simulink model "oloop1t"  (Simulink 2.09)
settings: Solver=ode15s  StartTime=0.0  StopTime=120  MaxStep=2  RelTol=1e-3  AbsTol=1e-3
undefined symbols (not defined in the file or in its folder): sfunyst, uaero0, uprop0
settings Model: SaveTime=off  SaveOutput=off  ConsistencyChecking=off  RTWTemplateMakefile=grt_vc.tmf

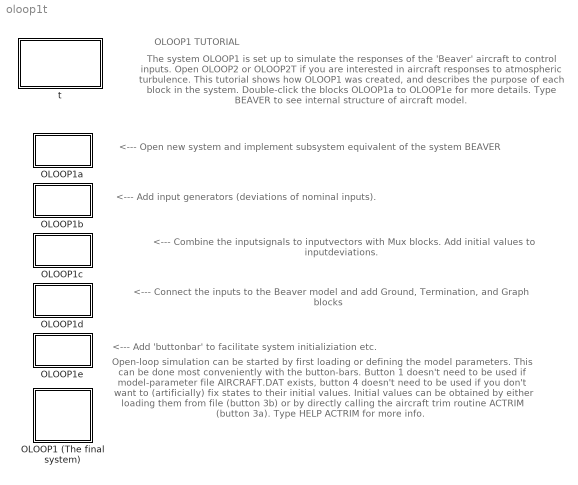
== system oloop1t ==
  note: OLOOP1 TUTORIAL
  note: <--- Connect the inputs to the Beaver model and add Ground, Termination, and Graph blocks
  note: <--- Combine the inputsignals to inputvectors with Mux blocks. Add initial values to inputdeviations.
  note: <--- Open new system and implement subsystem equivalent of the system BEAVER
  note: The system OLOOP1 is set up to simulate the responses of the 'Beaver' aircraft to control
      | inputs. Open OLOOP2 or OLOOP2T if you are interested in aircraft responses to
      | atmospheric turbulence. This tutorial shows how OLOOP1 was created, and describes
      | the purpose of each block in the system. Double-click the blocks OLOOP1a to OLOOP1e
      | for more details. Type BEAVER to see internal structure of aircraft model.
  note: <--- Add input generators (deviations of nominal inputs).
  note: Open-loop simulation can be started by first loading or defining the model parameters.
      | This can be done most conveniently with the button-bars. Button 1 doesn't need to
      | be used if model-parameter file AIRCRAFT.DAT exists, button 4 doesn't need to be
      |  used if you don't want to (artificially) fix states to their initial values. Initial values can be
      | obtained by either loading them from file (button 3b) or by directly calling the aircraft
      | trim routine ACTRIM (button 3a). Type HELP ACTRIM for more info.
  note: <--- Add 'buttonbar' to facilitate system initializiation etc.
  OLOOP1 (The final system) : Subsystem
      settings: OpenFcn=oloop1
  OLOOP1a : Subsystem
  OLOOP1b : Subsystem
  OLOOP1c : Subsystem
  OLOOP1d : Subsystem
  OLOOP1e : Subsystem
  t : Subsystem
      settings: OpenFcn=fdchelp oloop
      mask Display: disp('OLOOP1T\nMarc Rauw\nOctober 1997')

== system oloop1t/OLOOP1 (The final system) ==

== system oloop1t/OLOOP1a ==
  note: Construction of OLOOP1
  note: Step 1: open a new system
  note: Step 2: open the main FDC library FDCLIB by typing fdclib at the Matlab command-line
  note: Step 3: double-click the upper-right, light blue block (subsystem equivalents of the model BEAVER),
      | and copy the open-loop version of these subsystems to the new Simulink system
  note: Note: here a dummy version of  this
      | model has been used to reduce the
      | file-size of the tutorial
  Beaver model : Subsystem
  wires:
  Beaver model/1(V) -> ?
  Beaver model/2(alpha) -> ?
  Beaver model/3(beta) -> ?
  Beaver model/4(p) -> ?
  Beaver model/5(q) -> ?
  Beaver model/6(r) -> ?
  Beaver model/7(psi) -> ?
  Beaver model/8(theta) -> ?
  Beaver model/9(phi) -> ?
  Beaver model/10(xe) -> ?
  Beaver model/11(ye) -> ?
  Beaver model/12(H) -> ?
  Beaver model/13(H dot) -> ?
  Beaver model/14(pb/2V) -> ?
  Beaver model/15(qc/V) -> ?
  Beaver model/16(rb/2V) -> ?
  ? -> Beaver model/1(uaero)
  ? -> Beaver model/2(uprop)
  ? -> Beaver model/3(uwind)

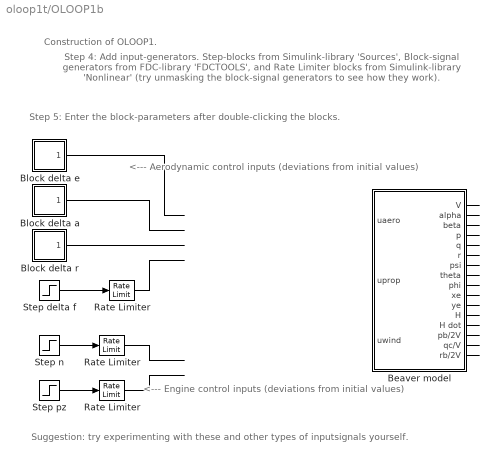
== system oloop1t/OLOOP1b ==
  note: Construction of OLOOP1.
  note: Step 5: Enter the block-parameters after double-clicking the blocks.
  note: Step 4: Add input-generators. Step-blocks from Simulink-library 'Sources', Block-signal generators
      | from FDC-library 'FDCTOOLS', and Rate Limiter blocks from Simulink-library 'Nonlinear'
      | (try unmasking the block-signal generators to see how they work).
  note: Suggestion: try experimenting with these and other types of inputsignals yourself.
  note: <--- Engine control inputs
      | (deviations from initial values)
  note: <--- Aerodynamic control inputs
      | (deviations from initial values)
  " Rate Limiter" : RateLimiter  RisingSlewLimit=1.0  FallingSlewLimit=-1.0
  Beaver model : Subsystem
  Block delta a : Subsystem  mask(Block Fcn){@1=0, @2=3*pi/180, @3=0, @4=2}
      mask prompts: @1 "Initial value (=final value):"; @2 "Amplitude of block (+ = step up, - = step down):"; @3 "Start time of block:"; @4 "Stop time of block:"
      mask help: Block Function
      mask init:
      | yinit=@1; yblock=@2; tstart=@3; tstop=@4;
      mask Help: This block implements a block signal.\nDefine the initial (=final) value, the\namplitude of the block (positive\n= upwards, negative=downwards),\nthe start time, and the stop time (must\nbe smaller than the start time).
      mask Display: plot(0,0,100,100,[100,60,60,20,20,0],[50,50,89,89,50,50])
  Block delta e : Subsystem  mask(Block Fcn){@1=0, @2=3*pi/180, @3=0, @4=2}
      mask prompts: @1 "Initial value (=final value):"; @2 "Amplitude of block (+ = step up, - = step down):"; @3 "Start time of block:"; @4 "Stop time of block:"
      mask help: Block Function
      mask init:
      | yinit=@1; yblock=@2; tstart=@3; tstop=@4;
      mask Help: This block implements a block signal.\nDefine the initial (=final) value, the\namplitude of the block (positive\n= upwards, negative=downwards),\nthe start time, and the stop time (must\nbe smaller than the start time).
      mask Display: plot(0,0,100,100,[100,60,60,20,20,0],[50,50,89,89,50,50])
  Block delta r : Subsystem  mask(Block Fcn){@1=0, @2=3*pi/180, @3=0, @4=2}
      mask prompts: @1 "Initial value (=final value):"; @2 "Amplitude of block (+ = step up, - = step down):"; @3 "Start time of block:"; @4 "Stop time of block:"
      mask help: Block Function
      mask init:
      | yinit=@1; yblock=@2; tstart=@3; tstop=@4;
      mask Help: This block implements a block signal.\nDefine the initial (=final) value, the\namplitude of the block (positive\n= upwards, negative=downwards),\nthe start time, and the stop time (must\nbe smaller than the start time).
      mask Display: plot(0,0,100,100,[100,60,60,20,20,0],[50,50,89,89,50,50])
  Rate Limiter : RateLimiter  RisingSlewLimit=3*pi/180  FallingSlewLimit=-3*pi/180
  "Rate Limiter " : RateLimiter  RisingSlewLimit=50  FallingSlewLimit=-50
  Step delta f : Step  Time=0.001  Before=0  After=3*pi/180
  Step n : Step  Time=1  Before=0  After=200
  Step pz : Step  Time=0.001  Before=0  After=2
  wires:
  Block delta a/1(block) -> ?
  Block delta r/1(block) -> ?
  Step delta f/1 -> Rate Limiter/1
  Step n/1 -> "Rate Limiter "/1
  Step pz/1 -> " Rate Limiter"/1
  Block delta e/1(block) -> ?
  Rate Limiter/1 -> ?
  "Rate Limiter "/1 -> ?
  " Rate Limiter"/1 -> ?
  Beaver model/1(V) -> ?
  Beaver model/2(alpha) -> ?
  Beaver model/3(beta) -> ?
  Beaver model/4(p) -> ?
  Beaver model/5(q) -> ?
  Beaver model/6(r) -> ?
  Beaver model/7(psi) -> ?
  Beaver model/8(theta) -> ?
  Beaver model/9(phi) -> ?
  Beaver model/10(xe) -> ?
  Beaver model/11(ye) -> ?
  Beaver model/12(H) -> ?
  Beaver model/13(H dot) -> ?
  Beaver model/14(pb/2V) -> ?
  Beaver model/15(qc/V) -> ?
  Beaver model/16(rb/2V) -> ?
  ? -> Beaver model/1(uaero)
  ? -> Beaver model/2(uprop)
  ? -> Beaver model/3(uwind)

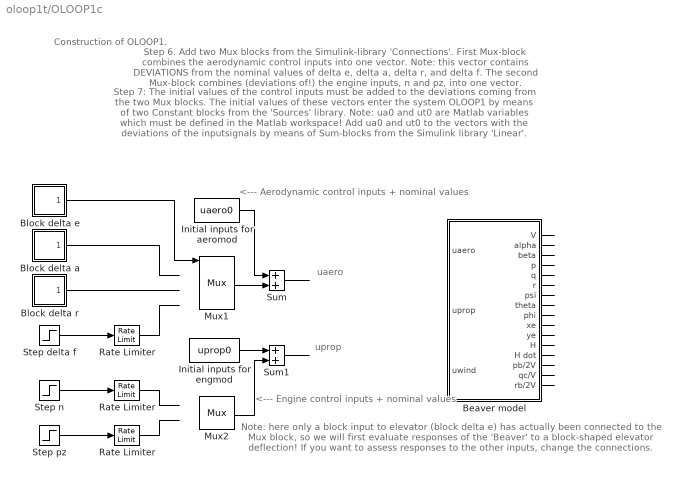
== system oloop1t/OLOOP1c ==
  note: uprop
  note: uaero
  note: Construction of OLOOP1.
  note: Note: here only a block input to elevator (block delta e) has actually
      | been connected to the Mux block, so we will first evaluate responses
      | of the 'Beaver' to a block-shaped elevator deflection! If you want to assess
      | responses to the other inputs, change the connections.
  note: <--- Aerodynamic control
      | inputs + nominal values
  note: <--- Engine control inputs +
      | nominal values
  note: Step 7: The initial values of the control inputs must be added to the deviations coming from the two Mux blocks. The initial
      | values of these vectors enter the system OLOOP1 by means of two Constant blocks from the 'Sources' library.
      | Note: ua0 and ut0 are Matlab variables which must be defined in the Matlab workspace! Add ua0 and ut0 to the
      | vectors with the deviations of the inputsignals by means of Sum-blocks from the Simulink library 'Linear'.
  note: Step 6. Add two Mux blocks from the Simulink-library 'Connections'. First Mux-block combines the aerodynamic control inputs
      | into one vector. Note: this vector contains DEVIATIONS from the nominal values of delta e, delta a, delta r, and delta f.
      | The second Mux-block combines (deviations of!) the engine inputs, n and pz, into one vector.
  " Rate Limiter" : RateLimiter  RisingSlewLimit=1.0  FallingSlewLimit=-1.0
  Beaver model : Subsystem
  Block delta a : Subsystem  mask(Block Fcn){@1=0, @2=3*pi/180, @3=0, @4=2}
      mask prompts: @1 "Initial value (=final value):"; @2 "Amplitude of block (+ = step up, - = step down):"; @3 "Start time of block:"; @4 "Stop time of block:"
      mask help: Block Function
      mask init:
      | yinit=@1; yblock=@2; tstart=@3; tstop=@4;
      mask Help: This block implements a block signal.\nDefine the initial (=final) value, the\namplitude of the block (positive\n= upwards, negative=downwards),\nthe start time, and the stop time (must\nbe smaller than the start time).
      mask Display: plot(0,0,100,100,[100,60,60,20,20,0],[50,50,89,89,50,50])
  Block delta e : Subsystem  mask(Block Fcn){@1=0, @2=3*pi/180, @3=0, @4=2}
      mask prompts: @1 "Initial value (=final value):"; @2 "Amplitude of block (+ = step up, - = step down):"; @3 "Start time of block:"; @4 "Stop time of block:"
      mask help: Block Function
      mask init:
      | yinit=@1; yblock=@2; tstart=@3; tstop=@4;
      mask Help: This block implements a block signal.\nDefine the initial (=final) value, the\namplitude of the block (positive\n= upwards, negative=downwards),\nthe start time, and the stop time (must\nbe smaller than the start time).
      mask Display: plot(0,0,100,100,[100,60,60,20,20,0],[50,50,89,89,50,50])
  Block delta r : Subsystem  mask(Block Fcn){@1=0, @2=3*pi/180, @3=0, @4=2}
      mask prompts: @1 "Initial value (=final value):"; @2 "Amplitude of block (+ = step up, - = step down):"; @3 "Start time of block:"; @4 "Stop time of block:"
      mask help: Block Function
      mask init:
      | yinit=@1; yblock=@2; tstart=@3; tstop=@4;
      mask Help: This block implements a block signal.\nDefine the initial (=final) value, the\namplitude of the block (positive\n= upwards, negative=downwards),\nthe start time, and the stop time (must\nbe smaller than the start time).
      mask Display: plot(0,0,100,100,[100,60,60,20,20,0],[50,50,89,89,50,50])
  Initial inputs for aeromod : Constant  Value=uaero0
  Initial inputs for engmod : Constant  Value=uprop0
  Mux1 : Mux  Inputs=4
  Mux2 : Mux  Inputs=2
  Rate Limiter : RateLimiter  RisingSlewLimit=3*pi/180  FallingSlewLimit=-3*pi/180
  "Rate Limiter " : RateLimiter  RisingSlewLimit=50  FallingSlewLimit=-50
  Step delta f : Step  Time=0.001  Before=0  After=3*pi/180
  Step n : Step  Time=1  Before=0  After=200
  Step pz : Step  Time=0.001  Before=0  After=2
  Sum : Sum  Inputs=++
  Sum1 : Sum  Inputs=++
  wires:
  Sum1/1 -> ?
  Sum/1 -> ?
  " Rate Limiter"/1 -> ?
  "Rate Limiter "/1 -> ?
  Rate Limiter/1 -> ?
  Block delta e/1(block) -> Mux1/1
  Step pz/1 -> " Rate Limiter"/1
  Step n/1 -> "Rate Limiter "/1
  Mux2/1 -> Sum1/2
  Mux1/1 -> Sum/2
  Initial inputs for aeromod/1 -> Sum/1
  Step delta f/1 -> Rate Limiter/1
  Initial inputs for engmod/1 -> Sum1/1
  Block delta r/1(block) -> ?
  Block delta a/1(block) -> ?
  Beaver model/2(alpha) -> ?
  Beaver model/3(beta) -> ?
  Beaver model/4(p) -> ?
  Beaver model/5(q) -> ?
  Beaver model/6(r) -> ?
  Beaver model/7(psi) -> ?
  Beaver model/8(theta) -> ?
  Beaver model/9(phi) -> ?
  Beaver model/10(xe) -> ?
  Beaver model/11(ye) -> ?
  Beaver model/12(H) -> ?
  Beaver model/13(H dot) -> ?
  Beaver model/14(pb/2V) -> ?
  Beaver model/15(qc/V) -> ?
  Beaver model/16(rb/2V) -> ?
  ? -> Beaver model/1(uaero)
  ? -> Beaver model/2(uprop)
  ? -> Beaver model/3(uwind)
  Beaver model/1(V) -> ?

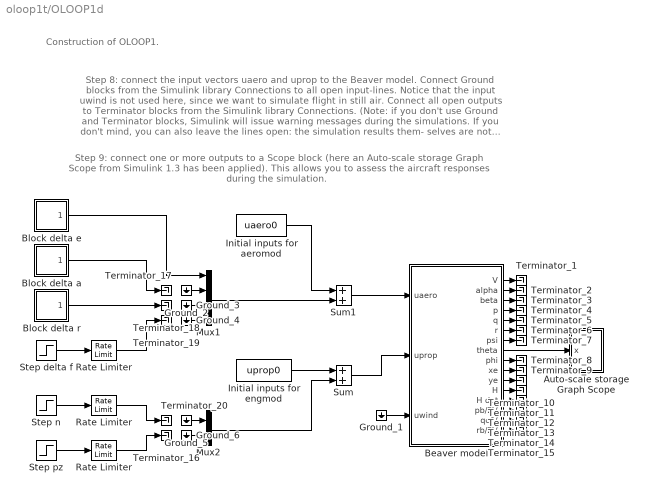
== system oloop1t/OLOOP1d ==
  note: Construction of OLOOP1.
  note: Step 9: connect one or more outputs to a Scope block (here an Auto-scale storage Graph Scope from
      | Simulink 1.3 has been applied). This allows you to assess the aircraft responses during the simulation.
  note: Step 8: connect the input vectors uaero and uprop to the Beaver model. Connect Ground blocks from the
      | Simulink library Connections to all open input-lines. Notice that the input uwind is not used here, since we
      | want to simulate flight in still air. Connect all open outputs to Terminator blocks from the Simulink library
      | Connections. (Note: if you don't use Ground and Terminator blocks, Simulink will issue warning messages
      | during the simulations. If you don't mind, you can also leave the lines open: the simulation results them-
      | selves are not affected by these warning messages).
  " Rate Limiter" : RateLimiter  RisingSlewLimit=1.0  FallingSlewLimit=-1.0
  Auto-scale storage Graph Scope : Subsystem  mask(Storage scope.){@1=5, @2=-0.02, @3=0.02, @4=200, @5='r-'}
      mask prompts: @1 "Initial Time Range:"; @2 "Initial y-min:"; @3 "Initial y-max:"; @4 "Storage pts.:"; @5 "Line type (rgbw-.:xo):"
      mask help:
      | Storage scope using MATLAB graph window.
      | Enter plotting ranges and line type.
      mask init:
      | npts = @4; color = @5; ax = [0, @1, @2, @3];
      mask Help: Uses MATLAB's graph window.\nUse only one block per system.\nLine type must be in quotes.\nSee the M-file sfunyst.m.
      mask Display: plot(0,0,100,100,[83,76,63,52,42,38,28,16,11,84,11,11,11,90,90,11],[75,58,47,54,72,80,84,74,65,65,65,90,40,40,90,90])
  Beaver model : Subsystem
  Block delta a : Subsystem  mask(Block Fcn){@1=0, @2=3*pi/180, @3=0, @4=2}
      mask prompts: @1 "Initial value (=final value):"; @2 "Amplitude of block (+ = step up, - = step down):"; @3 "Start time of block:"; @4 "Stop time of block:"
      mask help: Block Function
      mask init:
      | yinit=@1; yblock=@2; tstart=@3; tstop=@4;
      mask Help: This block implements a block signal.\nDefine the initial (=final) value, the\namplitude of the block (positive\n= upwards, negative=downwards),\nthe start time, and the stop time (must\nbe smaller than the start time).
      mask Display: plot(0,0,100,100,[100,60,60,20,20,0],[50,50,89,89,50,50])
  Block delta e : Subsystem  mask(Block Fcn){@1=0, @2=3*pi/180, @3=0, @4=2}
      mask prompts: @1 "Initial value (=final value):"; @2 "Amplitude of block (+ = step up, - = step down):"; @3 "Start time of block:"; @4 "Stop time of block:"
      mask help: Block Function
      mask init:
      | yinit=@1; yblock=@2; tstart=@3; tstop=@4;
      mask Help: This block implements a block signal.\nDefine the initial (=final) value, the\namplitude of the block (positive\n= upwards, negative=downwards),\nthe start time, and the stop time (must\nbe smaller than the start time).
      mask Display: plot(0,0,100,100,[100,60,60,20,20,0],[50,50,89,89,50,50])
  Block delta r : Subsystem  mask(Block Fcn){@1=0, @2=3*pi/180, @3=0, @4=2}
      mask prompts: @1 "Initial value (=final value):"; @2 "Amplitude of block (+ = step up, - = step down):"; @3 "Start time of block:"; @4 "Stop time of block:"
      mask help: Block Function
      mask init:
      | yinit=@1; yblock=@2; tstart=@3; tstop=@4;
      mask Help: This block implements a block signal.\nDefine the initial (=final) value, the\namplitude of the block (positive\n= upwards, negative=downwards),\nthe start time, and the stop time (must\nbe smaller than the start time).
      mask Display: plot(0,0,100,100,[100,60,60,20,20,0],[50,50,89,89,50,50])
  Ground_{1..6} (6 alike) : Ground
  Initial inputs for aeromod : Constant  Value=uaero0
  Initial inputs for engmod : Constant  Value=uprop0
  Mux1 : Mux  Inputs=4
  Mux2 : Mux  Inputs=2
  Rate Limiter : RateLimiter  RisingSlewLimit=3*pi/180  FallingSlewLimit=-3*pi/180
  "Rate Limiter " : RateLimiter  RisingSlewLimit=50  FallingSlewLimit=-50
  Step delta f : Step  Time=0.001  Before=0  After=3*pi/180
  Step n : Step  Time=1  Before=0  After=200
  Step pz : Step  Time=0.001  Before=0  After=2
  Sum : Sum  Inputs=++
  Sum1 : Sum  Inputs=++
  Terminator_{1..20} (20 alike) : Terminator
  wires:
  Beaver model/16(rb/2V) -> Terminator_15/1
  Beaver model/15(qc/V) -> Terminator_14/1
  Beaver model/14(pb/2V) -> Terminator_13/1
  Beaver model/13(H dot) -> Terminator_12/1
  Beaver model/12(H) -> Terminator_11/1
  Beaver model/11(ye) -> Terminator_10/1
  Beaver model/10(xe) -> Terminator_9/1
  Beaver model/9(phi) -> Terminator_8/1
  Beaver model/7(psi) -> Terminator_7/1
  Beaver model/6(r) -> Terminator_6/1
  Beaver model/5(q) -> Terminator_5/1
  Beaver model/4(p) -> Terminator_4/1
  Beaver model/3(beta) -> Terminator_3/1
  Beaver model/2(alpha) -> Terminator_2/1
  Beaver model/1(V) -> Terminator_1/1
  Mux2/1 -> Sum/2
  Initial inputs for aeromod/1 -> Sum1/1
  Sum/1 -> Beaver model/2(uprop)
  Initial inputs for engmod/1 -> Sum/1
  Sum1/1 -> Beaver model/1(uaero)
  Mux1/1 -> Sum1/2
  Ground_1/1 -> Beaver model/3(uwind)
  Block delta e/1(block) -> Mux1/1
  Step pz/1 -> " Rate Limiter"/1
  Step n/1 -> "Rate Limiter "/1
  Step delta f/1 -> Rate Limiter/1
  Ground_2/1 -> Mux1/2
  Ground_3/1 -> Mux1/3
  Ground_4/1 -> Mux1/4
  Ground_5/1 -> Mux2/1
  Ground_6/1 -> Mux2/2
  " Rate Limiter"/1 -> Terminator_16/1
  Block delta a/1(block) -> Terminator_17/1
  Block delta r/1(block) -> Terminator_18/1
  Rate Limiter/1 -> Terminator_19/1
  "Rate Limiter "/1 -> Terminator_20/1
  Beaver model/8(theta) -> Auto-scale storage Graph Scope/1(x)

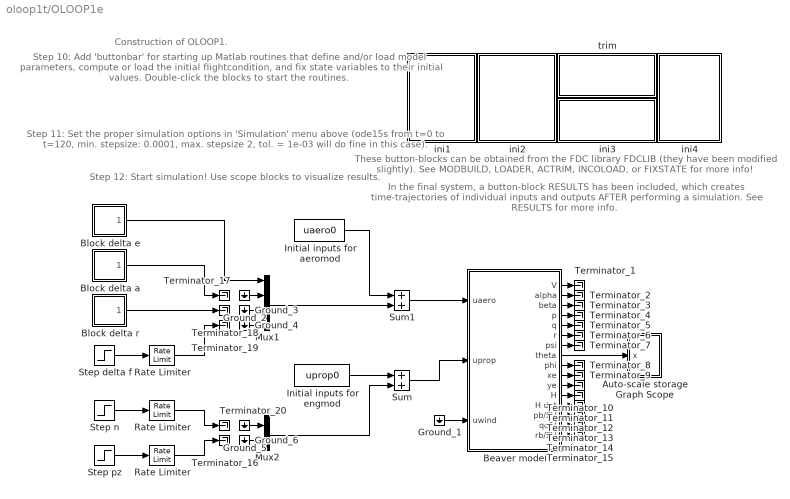
== system oloop1t/OLOOP1e ==
  note: Construction of OLOOP1.
  note: In the final system, a button-block RESULTS has been included,
      | which creates time-trajectories of individual inputs and outputs
      | AFTER performing a simulation. See RESULTS for more info.
  note: Step 11: Set the proper simulation options in 'Simulation' menu
      | above (ode15s from t=0 to t=120, min. stepsize: 0.0001,
      | max. stepsize 2, tol. = 1e-03 will do fine in this case).
  note: Step 12: Start simulation! Use scope blocks to visualize results.
  note: Step 10: Add 'buttonbar' for starting up Matlab routines that
      | define and/or load model parameters, compute or load the
      | initial flightcondition, and fix state variables to their initial
      | values. Double-click the blocks to start the routines.
  note: These button-blocks can be obtained from the FDC library
      | FDCLIB (they have been modified slightly). See MODBUILD,
      | LOADER, ACTRIM, INCOLOAD, or FIXSTATE for more info!
  " Rate Limiter" : RateLimiter  RisingSlewLimit=1.0  FallingSlewLimit=-1.0
  Auto-scale storage Graph Scope : Subsystem  mask(Storage scope.){@1=5, @2=-0.02, @3=0.02, @4=200, @5='r-'}
      mask prompts: @1 "Initial Time Range:"; @2 "Initial y-min:"; @3 "Initial y-max:"; @4 "Storage pts.:"; @5 "Line type (rgbw-.:xo):"
      mask help:
      | Storage scope using MATLAB graph window.
      | Enter plotting ranges and line type.
      mask init:
      | npts = @4; color = @5; ax = [0, @1, @2, @3];
      mask Help: Uses MATLAB's graph window.\nUse only one block per system.\nLine type must be in quotes.\nSee the M-file sfunyst.m.
      mask Display: plot(0,0,100,100,[83,76,63,52,42,38,28,16,11,84,11,11,11,90,90,11],[75,58,47,54,72,80,84,74,65,65,65,90,40,40,90,90])
  Beaver model : Subsystem
  Block delta a : Subsystem  mask(Block Fcn){@1=0, @2=3*pi/180, @3=0, @4=2}
      mask prompts: @1 "Initial value (=final value):"; @2 "Amplitude of block (+ = step up, - = step down):"; @3 "Start time of block:"; @4 "Stop time of block:"
      mask help: Block Function
      mask init:
      | yinit=@1; yblock=@2; tstart=@3; tstop=@4;
      mask Help: This block implements a block signal.\nDefine the initial (=final) value, the\namplitude of the block (positive\n= upwards, negative=downwards),\nthe start time, and the stop time (must\nbe smaller than the start time).
      mask Display: plot(0,0,100,100,[100,60,60,20,20,0],[50,50,89,89,50,50])
  Block delta e : Subsystem  mask(Block Fcn){@1=0, @2=3*pi/180, @3=0, @4=2}
      mask prompts: @1 "Initial value (=final value):"; @2 "Amplitude of block (+ = step up, - = step down):"; @3 "Start time of block:"; @4 "Stop time of block:"
      mask help: Block Function
      mask init:
      | yinit=@1; yblock=@2; tstart=@3; tstop=@4;
      mask Help: This block implements a block signal.\nDefine the initial (=final) value, the\namplitude of the block (positive\n= upwards, negative=downwards),\nthe start time, and the stop time (must\nbe smaller than the start time).
      mask Display: plot(0,0,100,100,[100,60,60,20,20,0],[50,50,89,89,50,50])
  Block delta r : Subsystem  mask(Block Fcn){@1=0, @2=3*pi/180, @3=0, @4=2}
      mask prompts: @1 "Initial value (=final value):"; @2 "Amplitude of block (+ = step up, - = step down):"; @3 "Start time of block:"; @4 "Stop time of block:"
      mask help: Block Function
      mask init:
      | yinit=@1; yblock=@2; tstart=@3; tstop=@4;
      mask Help: This block implements a block signal.\nDefine the initial (=final) value, the\namplitude of the block (positive\n= upwards, negative=downwards),\nthe start time, and the stop time (must\nbe smaller than the start time).
      mask Display: plot(0,0,100,100,[100,60,60,20,20,0],[50,50,89,89,50,50])
  Ground_{1..6} (6 alike) : Ground
  Initial inputs for aeromod : Constant  Value=uaero0
  Initial inputs for engmod : Constant  Value=uprop0
  Mux1 : Mux  Inputs=4
  Mux2 : Mux  Inputs=2
  Rate Limiter : RateLimiter  RisingSlewLimit=3*pi/180  FallingSlewLimit=-3*pi/180
  "Rate Limiter " : RateLimiter  RisingSlewLimit=50  FallingSlewLimit=-50
  Step delta f : Step  Time=0.001  Before=0  After=3*pi/180
  Step n : Step  Time=1  Before=0  After=200
  Step pz : Step  Time=0.001  Before=0  After=2
  Sum : Sum  Inputs=++
  Sum1 : Sum  Inputs=++
  Terminator_{1..20} (20 alike) : Terminator
  ini1 : Subsystem
      settings: OpenFcn=modbuild
      mask Type: modbuild
      mask Display: disp('(1). Create\ndatafiles\n\n\nMODBUILD')
  ini2 : Subsystem
      settings: OpenFcn=loader
      mask Type: loader
      mask Display: disp('2. Load model\nparameters\nfrom file\n\nLOADER')
  ini3 : Subsystem
      settings: OpenFcn=incoload
      mask Type: incoload
      mask Display: disp('3b. Load initial\ncondition from file\nINCOLOAD')
  ini4 : Subsystem
      settings: OpenFcn=fixstate
      mask Type: fixstate
      mask Display: disp('(4). Fix\nindividual\nstates\n\nFIXSTATE')
  trim : Subsystem
      settings: OpenFcn=actrim
      mask Type: aircraft trim
      mask Display: disp('3a. Call aircraft\ntrim routine\nACTRIM')
  wires:
  Beaver model/16(rb/2V) -> Terminator_15/1
  Beaver model/15(qc/V) -> Terminator_14/1
  Beaver model/14(pb/2V) -> Terminator_13/1
  Beaver model/13(H dot) -> Terminator_12/1
  Beaver model/12(H) -> Terminator_11/1
  Beaver model/11(ye) -> Terminator_10/1
  Beaver model/10(xe) -> Terminator_9/1
  Beaver model/9(phi) -> Terminator_8/1
  Beaver model/7(psi) -> Terminator_7/1
  Beaver model/6(r) -> Terminator_6/1
  Beaver model/5(q) -> Terminator_5/1
  Beaver model/4(p) -> Terminator_4/1
  Beaver model/3(beta) -> Terminator_3/1
  Beaver model/2(alpha) -> Terminator_2/1
  Beaver model/1(V) -> Terminator_1/1
  Mux2/1 -> Sum/2
  Initial inputs for aeromod/1 -> Sum1/1
  Sum/1 -> Beaver model/2(uprop)
  Initial inputs for engmod/1 -> Sum/1
  Sum1/1 -> Beaver model/1(uaero)
  Mux1/1 -> Sum1/2
  Ground_1/1 -> Beaver model/3(uwind)
  Block delta e/1(block) -> Mux1/1
  Step pz/1 -> " Rate Limiter"/1
  Step n/1 -> "Rate Limiter "/1
  Step delta f/1 -> Rate Limiter/1
  Ground_2/1 -> Mux1/2
  Ground_3/1 -> Mux1/3
  Ground_4/1 -> Mux1/4
  Ground_5/1 -> Mux2/1
  Ground_6/1 -> Mux2/2
  " Rate Limiter"/1 -> Terminator_16/1
  Block delta a/1(block) -> Terminator_17/1
  Block delta r/1(block) -> Terminator_18/1
  Rate Limiter/1 -> Terminator_19/1
  "Rate Limiter "/1 -> Terminator_20/1
  Beaver model/8(theta) -> Auto-scale storage Graph Scope/1(x)

== system oloop1t/t ==

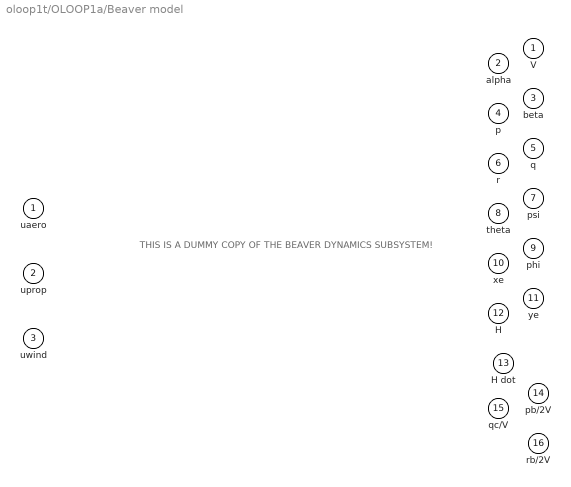
== system oloop1t/OLOOP1a/Beaver model ==
  note: THIS IS A DUMMY COPY
      | OF THE BEAVER
      | DYNAMICS SUBSYSTEM!
  uaero : Inport  Port=1  PortWidth=4  SampleTime=-1
  uprop : Inport  Port=2  PortWidth=2  SampleTime=-1
  uwind : Inport  Port=3  PortWidth=6  SampleTime=-1
  V : Outport  Port=1  InitialOutput=0
  alpha : Outport  Port=2  InitialOutput=0
  beta : Outport  Port=3  InitialOutput=0
  p : Outport  Port=4  InitialOutput=0
  q : Outport  Port=5  InitialOutput=0
  r : Outport  Port=6  InitialOutput=0
  psi : Outport  Port=7  InitialOutput=0
  theta : Outport  Port=8  InitialOutput=0
  phi : Outport  Port=9  InitialOutput=0
  xe : Outport  Port=10  InitialOutput=0
  ye : Outport  Port=11  InitialOutput=0
  H : Outport  Port=12  InitialOutput=0
  H dot : Outport  Port=13  InitialOutput=0
  pb/2V : Outport  Port=14  InitialOutput=0
  qc/V : Outport  Port=15  InitialOutput=0
  rb/2V : Outport  Port=16  InitialOutput=0

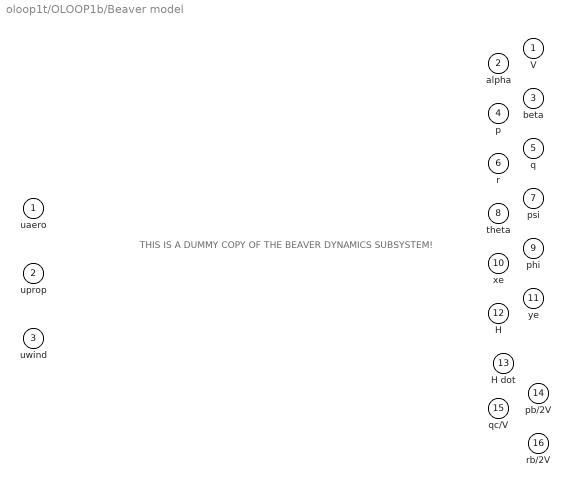
== system oloop1t/OLOOP1b/Beaver model ==
  note: THIS IS A DUMMY COPY
      | OF THE BEAVER
      | DYNAMICS SUBSYSTEM!
  uaero : Inport  Port=1  PortWidth=4  SampleTime=-1
  uprop : Inport  Port=2  PortWidth=2  SampleTime=-1
  uwind : Inport  Port=3  PortWidth=6  SampleTime=-1
  V : Outport  Port=1  InitialOutput=0
  alpha : Outport  Port=2  InitialOutput=0
  beta : Outport  Port=3  InitialOutput=0
  p : Outport  Port=4  InitialOutput=0
  q : Outport  Port=5  InitialOutput=0
  r : Outport  Port=6  InitialOutput=0
  psi : Outport  Port=7  InitialOutput=0
  theta : Outport  Port=8  InitialOutput=0
  phi : Outport  Port=9  InitialOutput=0
  xe : Outport  Port=10  InitialOutput=0
  ye : Outport  Port=11  InitialOutput=0
  H : Outport  Port=12  InitialOutput=0
  H dot : Outport  Port=13  InitialOutput=0
  pb/2V : Outport  Port=14  InitialOutput=0
  qc/V : Outport  Port=15  InitialOutput=0
  rb/2V : Outport  Port=16  InitialOutput=0

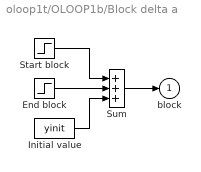
== system oloop1t/OLOOP1b/Block delta a ==
  End block : Step  Time=tstop  Before=0  After=-yblock
  Initial value : Constant  Value=yinit
  Start block : Step  Time=tstart  Before=0  After=yblock
  Sum : Sum  Inputs=+++
  block : Outport  Port=1  InitialOutput=0
  wires:
  Sum/1 -> block/1
  Initial value/1 -> Sum/3
  Start block/1 -> Sum/1
  End block/1 -> Sum/2

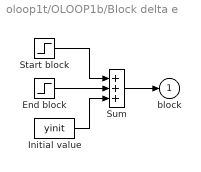
== system oloop1t/OLOOP1b/Block delta e ==
  End block : Step  Time=tstop  Before=0  After=-yblock
  Initial value : Constant  Value=yinit
  Start block : Step  Time=tstart  Before=0  After=yblock
  Sum : Sum  Inputs=+++
  block : Outport  Port=1  InitialOutput=0
  wires:
  End block/1 -> Sum/2
  Start block/1 -> Sum/1
  Initial value/1 -> Sum/3
  Sum/1 -> block/1

== system oloop1t/OLOOP1b/Block delta r ==
  End block : Step  Time=tstop  Before=0  After=-yblock
  Initial value : Constant  Value=yinit
  Start block : Step  Time=tstart  Before=0  After=yblock
  Sum : Sum  Inputs=+++
  block : Outport  Port=1  InitialOutput=0
  wires:
  End block/1 -> Sum/2
  Start block/1 -> Sum/1
  Initial value/1 -> Sum/3
  Sum/1 -> block/1

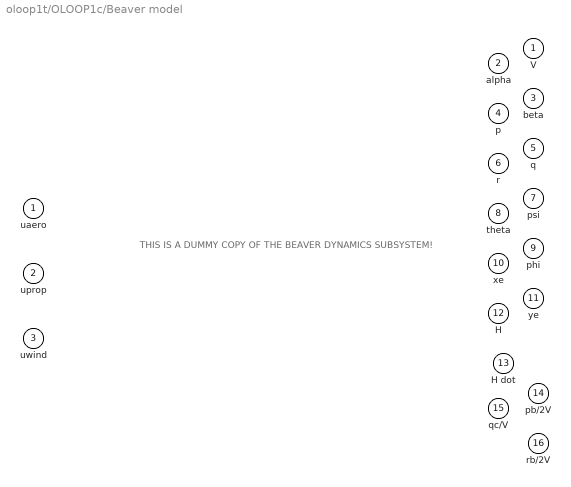
== system oloop1t/OLOOP1c/Beaver model ==
  note: THIS IS A DUMMY COPY
      | OF THE BEAVER
      | DYNAMICS SUBSYSTEM!
  uaero : Inport  Port=1  PortWidth=4  SampleTime=-1
  uprop : Inport  Port=2  PortWidth=2  SampleTime=-1
  uwind : Inport  Port=3  PortWidth=6  SampleTime=-1
  V : Outport  Port=1  InitialOutput=0
  alpha : Outport  Port=2  InitialOutput=0
  beta : Outport  Port=3  InitialOutput=0
  p : Outport  Port=4  InitialOutput=0
  q : Outport  Port=5  InitialOutput=0
  r : Outport  Port=6  InitialOutput=0
  psi : Outport  Port=7  InitialOutput=0
  theta : Outport  Port=8  InitialOutput=0
  phi : Outport  Port=9  InitialOutput=0
  xe : Outport  Port=10  InitialOutput=0
  ye : Outport  Port=11  InitialOutput=0
  H : Outport  Port=12  InitialOutput=0
  H dot : Outport  Port=13  InitialOutput=0
  pb/2V : Outport  Port=14  InitialOutput=0
  qc/V : Outport  Port=15  InitialOutput=0
  rb/2V : Outport  Port=16  InitialOutput=0

== system oloop1t/OLOOP1c/Block delta a ==
  End block : Step  Time=tstop  Before=0  After=-yblock
  Initial value : Constant  Value=yinit
  Start block : Step  Time=tstart  Before=0  After=yblock
  Sum : Sum  Inputs=+++
  block : Outport  Port=1  InitialOutput=0
  wires:
  Sum/1 -> block/1
  Initial value/1 -> Sum/3
  Start block/1 -> Sum/1
  End block/1 -> Sum/2

== system oloop1t/OLOOP1c/Block delta e ==
  End block : Step  Time=tstop  Before=0  After=-yblock
  Initial value : Constant  Value=yinit
  Start block : Step  Time=tstart  Before=0  After=yblock
  Sum : Sum  Inputs=+++
  block : Outport  Port=1  InitialOutput=0
  wires:
  End block/1 -> Sum/2
  Start block/1 -> Sum/1
  Initial value/1 -> Sum/3
  Sum/1 -> block/1

== system oloop1t/OLOOP1c/Block delta r ==
  End block : Step  Time=tstop  Before=0  After=-yblock
  Initial value : Constant  Value=yinit
  Start block : Step  Time=tstart  Before=0  After=yblock
  Sum : Sum  Inputs=+++
  block : Outport  Port=1  InitialOutput=0
  wires:
  End block/1 -> Sum/2
  Start block/1 -> Sum/1
  Initial value/1 -> Sum/3
  Sum/1 -> block/1

== system oloop1t/OLOOP1d/Auto-scale storage Graph Scope ==
  x : Inport  Port=1  PortWidth=-1  SampleTime=-1
  "S-function M-file which plots lines " : S-Function  LoadFcn=sfunyst([],[],[],'LoadBlock')  FunctionName=sfunyst  Parameters=ax, color, npts
      settings: CopyFcn=sfunyst([],[],[],'CopyBlock')  DeleteFcn=sfunyst([],[],[],'DeleteBlock')
  wires:
  x/1 -> "S-function M-file which plots lines "/1

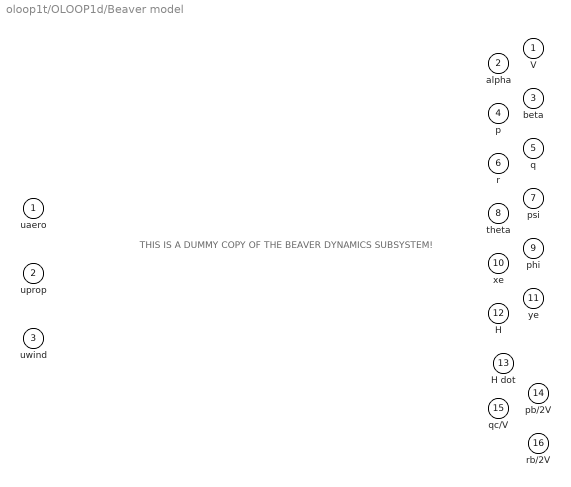
== system oloop1t/OLOOP1d/Beaver model ==
  note: THIS IS A DUMMY COPY
      | OF THE BEAVER
      | DYNAMICS SUBSYSTEM!
  uaero : Inport  Port=1  PortWidth=4  SampleTime=-1
  uprop : Inport  Port=2  PortWidth=2  SampleTime=-1
  uwind : Inport  Port=3  PortWidth=6  SampleTime=-1
  V : Outport  Port=1  InitialOutput=0
  alpha : Outport  Port=2  InitialOutput=0
  beta : Outport  Port=3  InitialOutput=0
  p : Outport  Port=4  InitialOutput=0
  q : Outport  Port=5  InitialOutput=0
  r : Outport  Port=6  InitialOutput=0
  psi : Outport  Port=7  InitialOutput=0
  theta : Outport  Port=8  InitialOutput=0
  phi : Outport  Port=9  InitialOutput=0
  xe : Outport  Port=10  InitialOutput=0
  ye : Outport  Port=11  InitialOutput=0
  H : Outport  Port=12  InitialOutput=0
  H dot : Outport  Port=13  InitialOutput=0
  pb/2V : Outport  Port=14  InitialOutput=0
  qc/V : Outport  Port=15  InitialOutput=0
  rb/2V : Outport  Port=16  InitialOutput=0

== system oloop1t/OLOOP1d/Block delta a ==
  End block : Step  Time=tstop  Before=0  After=-yblock
  Initial value : Constant  Value=yinit
  Start block : Step  Time=tstart  Before=0  After=yblock
  Sum : Sum  Inputs=+++
  block : Outport  Port=1  InitialOutput=0
  wires:
  End block/1 -> Sum/2
  Start block/1 -> Sum/1
  Initial value/1 -> Sum/3
  Sum/1 -> block/1

== system oloop1t/OLOOP1d/Block delta e ==
  End block : Step  Time=tstop  Before=0  After=-yblock
  Initial value : Constant  Value=yinit
  Start block : Step  Time=tstart  Before=0  After=yblock
  Sum : Sum  Inputs=+++
  block : Outport  Port=1  InitialOutput=0
  wires:
  Sum/1 -> block/1
  Initial value/1 -> Sum/3
  Start block/1 -> Sum/1
  End block/1 -> Sum/2

== system oloop1t/OLOOP1d/Block delta r ==
  End block : Step  Time=tstop  Before=0  After=-yblock
  Initial value : Constant  Value=yinit
  Start block : Step  Time=tstart  Before=0  After=yblock
  Sum : Sum  Inputs=+++
  block : Outport  Port=1  InitialOutput=0
  wires:
  Sum/1 -> block/1
  Initial value/1 -> Sum/3
  Start block/1 -> Sum/1
  End block/1 -> Sum/2

== system oloop1t/OLOOP1e/Auto-scale storage Graph Scope ==
  x : Inport  Port=1  PortWidth=-1  SampleTime=-1
  "S-function M-file which plots lines " : S-Function  LoadFcn=sfunyst([],[],[],'LoadBlock')  FunctionName=sfunyst  Parameters=ax, color, npts
      settings: CopyFcn=sfunyst([],[],[],'CopyBlock')  DeleteFcn=sfunyst([],[],[],'DeleteBlock')
  wires:
  x/1 -> "S-function M-file which plots lines "/1

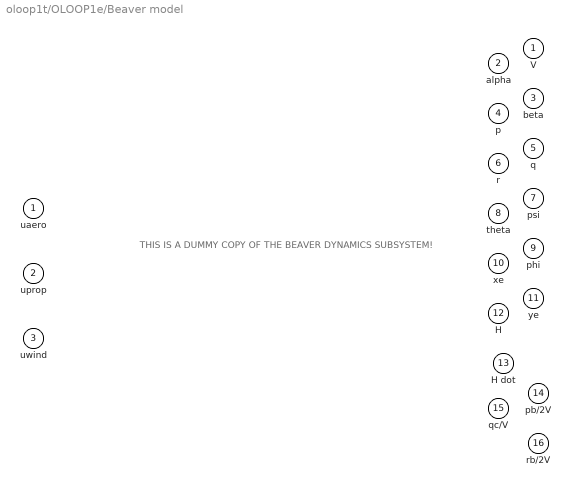
== system oloop1t/OLOOP1e/Beaver model ==
  note: THIS IS A DUMMY COPY
      | OF THE BEAVER
      | DYNAMICS SUBSYSTEM!
  uaero : Inport  Port=1  PortWidth=4  SampleTime=-1
  uprop : Inport  Port=2  PortWidth=2  SampleTime=-1
  uwind : Inport  Port=3  PortWidth=6  SampleTime=-1
  V : Outport  Port=1  InitialOutput=0
  alpha : Outport  Port=2  InitialOutput=0
  beta : Outport  Port=3  InitialOutput=0
  p : Outport  Port=4  InitialOutput=0
  q : Outport  Port=5  InitialOutput=0
  r : Outport  Port=6  InitialOutput=0
  psi : Outport  Port=7  InitialOutput=0
  theta : Outport  Port=8  InitialOutput=0
  phi : Outport  Port=9  InitialOutput=0
  xe : Outport  Port=10  InitialOutput=0
  ye : Outport  Port=11  InitialOutput=0
  H : Outport  Port=12  InitialOutput=0
  H dot : Outport  Port=13  InitialOutput=0
  pb/2V : Outport  Port=14  InitialOutput=0
  qc/V : Outport  Port=15  InitialOutput=0
  rb/2V : Outport  Port=16  InitialOutput=0

== system oloop1t/OLOOP1e/Block delta a ==
  End block : Step  Time=tstop  Before=0  After=-yblock
  Initial value : Constant  Value=yinit
  Start block : Step  Time=tstart  Before=0  After=yblock
  Sum : Sum  Inputs=+++
  block : Outport  Port=1  InitialOutput=0
  wires:
  End block/1 -> Sum/2
  Start block/1 -> Sum/1
  Initial value/1 -> Sum/3
  Sum/1 -> block/1

== system oloop1t/OLOOP1e/Block delta e ==
  End block : Step  Time=tstop  Before=0  After=-yblock
  Initial value : Constant  Value=yinit
  Start block : Step  Time=tstart  Before=0  After=yblock
  Sum : Sum  Inputs=+++
  block : Outport  Port=1  InitialOutput=0
  wires:
  Sum/1 -> block/1
  Initial value/1 -> Sum/3
  Start block/1 -> Sum/1
  End block/1 -> Sum/2

== system oloop1t/OLOOP1e/Block delta r ==
  End block : Step  Time=tstop  Before=0  After=-yblock
  Initial value : Constant  Value=yinit
  Start block : Step  Time=tstart  Before=0  After=yblock
  Sum : Sum  Inputs=+++
  block : Outport  Port=1  InitialOutput=0
  wires:
  Sum/1 -> block/1
  Initial value/1 -> Sum/3
  Start block/1 -> Sum/1
  End block/1 -> Sum/2

== system oloop1t/OLOOP1e/ini1 ==

== system oloop1t/OLOOP1e/ini2 ==

== system oloop1t/OLOOP1e/ini3 ==

== system oloop1t/OLOOP1e/ini4 ==

== system oloop1t/OLOOP1e/trim ==
  note: This block is used to set the initial values of the
      | state variables of the aircraft model.
      |
      | x = [V alpha beta p q r psi theta phi xe ye H]'
      |
      | x0 is stored in the file EQMINCO.mat and loaded
      | by the integrator block of the aircraft model.
